simulink model "ISReferenceApplication"  (R2019b)
settings: Solver=VariableStepAuto  StartTime=0.0  StopTime=10.0  RelTol=1e-3
undefined symbols (not defined in the file or in its folder): C_Brake, C_Final, C_Front, C_Middle, C_out_Brake, C_out_Final, C_out_Front, C_out_Middle, Co, Cso, D_out_Brake, D_out_Final, D_out_Front, D_out_Middle, Downshift_Speeds, F, F_Brake, F_Final, F_Front, F_Middle, Fs, G_Brake, G_Final, G_Front, G_Middle, G_sys_Brake, G_sys_Final, G_sys_Front, G_sys_Middle, Gd, Gd_Brake, Gd_Final, Gsd, h, H_Brake, H_Final, H_Front, H_Middle, H_sys_Brake, H_sys_Final, H_sys_Front, H_sys_Middle, Hd, Hd_Brake, Hd_Final, Hsd, JE, JE_Brake, JE_Final, JE_Front, JE_Middle, JEs, JF_part, JF_part_Brake, JF_part_Final, JF_parts, Ld, Ld_Brake, Ld_Final, Ld_Front ... (+21)
libraries: simulink x5, autolibutils x3, sim3dlib x2, vehdynlibviscommon x1
(part 1 of 4)
settings Model: Creator=User  LastModifiedBy=User

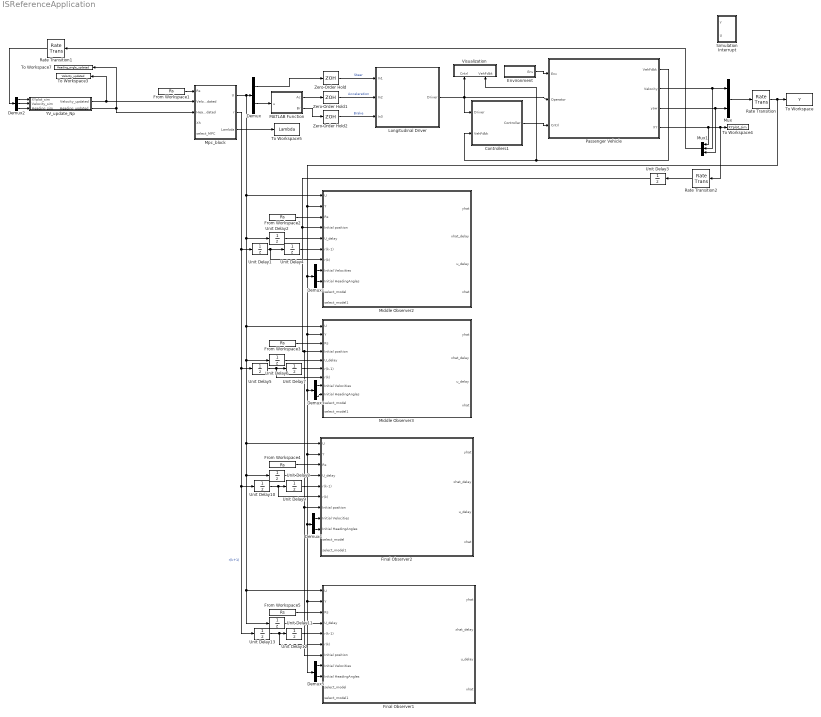
== system ISReferenceApplication ==
  Controllers1 : Subsystem
      mask Display: image('SystemControllers.png')
  Demux{,1,3..5} (5 alike) : Demux  Outputs=2
  Demux2 : Demux  Outputs=3
  Environment : Subsystem  TreatAsAtomicUnit=on
      mask Display: disp('Environment')
  Final Observer1 : Subsystem
  Final Observer2 : Subsystem
  From Workspace{1..5} (5 alike) : FromWorkspace  VariableName=Rs  SampleTime=Ts
  Longitudinal Driver : Subsystem  SystemSampleTime=Tf  VariantControl=0
      mask Display: image('longitudinal_driver_pedals.png');
  MATLAB Function : MATLAB Function  TreatAsAtomicUnit=on  SystemSampleTime=Ts
  Middle Observer2 : Subsystem
  Middle Observer3 : Subsystem
  Mpc_block : Subsystem  TreatAsAtomicUnit=on  SystemSampleTime=Ts
  Mux : Mux  Inputs=2
  Mux1 : Mux  Inputs=3
  Passenger Vehicle : Subsystem
      mask Display: image('PassengerVehicle.png')
  Rate Transition : RateTransition  OutPortSampleTime=Ts
  Rate Transition1 : RateTransition  OutPortSampleTime=Ts
  Rate Transition2 : RateTransition  OutPortSampleTime=Ts
  "Simulation Interrupt " : Subsystem
  To Workspace : ToWorkspace  VariableName=Y  SampleTime=Ts
  To Workspace3 : ToWorkspace  VariableName=Velocity_updated  SampleTime=Ts
      settings: Save2DSignal=2-D array (concatenate along first dimension)
  To Workspace4 : ToWorkspace  VariableName=XYplot_sim  SampleTime=Ts
  To Workspace5 : ToWorkspace  VariableName=Lambda  SampleTime=Ts
  To Workspace7 : ToWorkspace  VariableName=Heading_angle_updated  SampleTime=Ts
      settings: Save2DSignal=2-D array (concatenate along first dimension)
  Unit Delay{1..13} (13 alike) : UnitDelay  SampleTime=Ts  HasFrameUpgradeWarning=on
  Visualization : Subsystem  TreatAsAtomicUnit=on
      mask Display: disp('Visualization')
  YV_update_Np : Subsystem  TreatAsAtomicUnit=on
  Zero-Order Hold : ZeroOrderHold  SampleTime=Tf
  Zero-Order Hold1 : ZeroOrderHold  SampleTime=Tf
  Zero-Order Hold2 : ZeroOrderHold  SampleTime=Tf
  wires:
  Controllers1/1(Controller) -> Passenger Vehicle/3(Cntrl)
  Longitudinal Driver/1(Driver) -> Visualization/1(Cntrl), Controllers1/1(Driver), Passenger Vehicle/2(Operator)
  Environment/1(Env) -> Passenger Vehicle/1(Env)
  Passenger Vehicle/1(VehFdbk) -> Visualization/2(VehFdbk), Controllers1/2(VehFdbk)
  Zero-Order Hold2/1 -> Longitudinal Driver/3(In3)  "Brake"
  Zero-Order Hold1/1 -> Longitudinal Driver/2(In2)  "Acceleration"
  Zero-Order Hold/1 -> Longitudinal Driver/1(In1)  "Steer"
  MATLAB Function/1(Ac) -> Zero-Order Hold1/1
  MATLAB Function/2(Br) -> Zero-Order Hold2/1
  Demux/2 -> MATLAB Function/1(u)
  Demux/1 -> Zero-Order Hold/1
  Mpc_block/1(U) -> Middle Observer2/1(U), Unit Delay11/1, Final Observer1/1(U), Unit Delay8/1, Final Observer2/1(U), Unit Delay6/1, Middle Observer3/1(U), Unit Delay2/1, Demux/1
  Mpc_block/3(Lambda) -> To Workspace5/1
  From Workspace1/1 -> Mpc_block/1(Rs)
  YV_update_Np/1(Velocity_updated) -> To Workspace3/1, Mpc_block/2(Velocity_updated)
  YV_update_Np/2(Heading_updated) -> To Workspace7/1, Mpc_block/3(Heading_updated)
  Demux2/1 -> YV_update_Np/1(XYplot_sim)
  Demux2/2 -> YV_update_Np/2(Velocity_sim)
  Demux2/3 -> YV_update_Np/3(Heading_sim)
  Rate Transition1/1 -> Demux2/1
  Mux/1 -> Rate Transition/1
  Passenger Vehicle/2(Velocity) -> Mux1/2, Mux/1
  Passenger Vehicle/3(yaw) -> Mux1/3, Mux/2
  Passenger Vehicle/4(XY) -> Mux1/1, Rate Transition2/1, To Workspace4/1
  Rate Transition/1 -> Final Observer2/2(Y), Final Observer1/2(Y), Demux5/1, Demux4/1, Demux3/1, Middle Observer3/2(Y), Demux1/1, Middle Observer2/2(Y), To Workspace/1
  Mux1/1 -> Rate Transition1/1
  Rate Transition2/1 -> Unit Delay3/1
  Unit Delay3/1 -> Final Observer1/7(Initial position), Final Observer2/7(Initial position), Middle Observer3/4(Initial position), Middle Observer2/4(Initial position)
  Unit Delay2/1 -> Middle Observer2/5(U_delay)
  Unit Delay4/1 -> Middle Observer2/6(r(k-1))
  Unit Delay1/1 -> Middle Observer2/7(r(k)), Unit Delay4/1
  Mpc_block/2(r) -> Unit Delay13/1, Unit Delay10/1, Unit Delay5/1, Unit Delay1/1  "r(k+1)"
  From Workspace2/1 -> Middle Observer2/3(Rs)
  Demux1/1 -> Middle Observer2/8(Initial Velocities)
  Demux1/2 -> Middle Observer2/9(Initial HeadingAngles)
  Unit Delay6/1 -> Middle Observer3/5(U_delay)
  Unit Delay7/1 -> Middle Observer3/6(r(k-1))
  Unit Delay5/1 -> Middle Observer3/7(r(k)), Unit Delay7/1
  From Workspace3/1 -> Middle Observer3/3(Rs)
  Demux3/1 -> Middle Observer3/8(Initial Velocities)
  Demux3/2 -> Middle Observer3/9(Initial HeadingAngles)
  From Workspace4/1 -> Final Observer2/3(Rs)
  Unit Delay8/1 -> Final Observer2/4(U_delay)
  Unit Delay9/1 -> Final Observer2/5(r(k-1))
  Unit Delay10/1 -> Final Observer2/6(r(k)), Unit Delay9/1
  Demux4/1 -> Final Observer2/8(Initial Velocities)
  Demux4/2 -> Final Observer2/9(Initial HeadingAngles)
  From Workspace5/1 -> Final Observer1/3(Rs)
  Unit Delay11/1 -> Final Observer1/4(U_delay)
  Unit Delay12/1 -> Final Observer1/5(r(k-1))
  Unit Delay13/1 -> Final Observer1/6(r(k)), Unit Delay12/1
  Demux5/1 -> Final Observer1/8(Initial Velocities)
  Demux5/2 -> Final Observer1/9(Initial HeadingAngles)

== system ISReferenceApplication/Controllers1 ==
  Driver : Inport
  VehFdbk : Inport  Port=2
  Active Differential Control : Subsystem  VariantControlMode=Label  Variant=on  LabelModeActiveChoice=0
  Brake Controller : Subsystem
  Bus Creator{,1..2,4} (4 alike) : BusCreator  Inputs=1
  Bus Creator3 : BusCreator  Inputs=4
  Bus Selector : BusSelector  OutputSignals=Body.xdot,Wheels.Kappa,Body.r
  Bus Selector1 : BusSelector  OutputSignals=Driveline.EngSpd,Driveline.PropShftSpd
  Bus Selector2 : BusSelector  OutputSignals=AccelCmd,DecelCmd
  Bus Selector3 : BusSelector  OutputSignals=SteerCmd
  ECU : Subsystem
  Max : MinMax  Function=max  Inputs=2
  Transmission Controller : Subsystem
  Controller : Outport  VectorParamsAs1DForOutWhenUnconnected=off
  wires:
  Bus Selector/3 -> Active Differential Control/1(YawRate)  "<r>"
  [DiffTrqCmd] -> Max/2
  Max/1 -> Bus Creator/1  "EngTrqCmd"
  Active Differential Control/2(TrqCmd) -> [DiffTrqCmd]
  Bus Selector3/1 -> Active Differential Control/2(Steer)  "<SteerCmd>"
  Active Differential Control/1(DiffPrsCmd) -> Bus Creator4/1  "DiffPrsCmd"
  Bus Creator4/1 -> Bus Creator3/4  "Diff"
  Bus Creator3/1 -> Controller/1  "Controller"
  Bus Creator2/1 -> Bus Creator3/3  "Brake"
  Bus Creator1/1 -> Bus Creator3/2  "Transmission"
  Bus Creator/1 -> Bus Creator3/1  "ECU"
  Bus Selector2/2 -> Brake Controller/1(BrkCmd)  "<DecelCmd>"
  Bus Selector2/1 -> ECU/1(<Accel>), Transmission Controller/1(Acc)  "<AccelCmd>"
  Driver/1 -> Bus Selector2/1, Bus Selector3/1
  Bus Selector1/2 -> Transmission Controller/3(PropShaftSpd)  "<PropShftSpd>"
  Bus Selector1/1 -> Transmission Controller/2(EngSpd)  "<EngSpd>"
  Bus Selector/1 -> Brake Controller/2(xdot)  "<xdot>"
  VehFdbk/1 -> Bus Selector1/1, Bus Selector/1
  Brake Controller/1(PCmd) -> Bus Creator2/1  "BrkPrsCmd"
  ECU/1(Trq Cmd) -> Max/1
  Bus Selector/2 -> Brake Controller/3(kappa)  "<Kappa>"
  Transmission Controller/1(Gear) -> Bus Creator1/1  "GearCmd"

== system ISReferenceApplication/Environment ==
  Bus Creator : BusCreator  Inputs=4
  Bus Creator1 : BusCreator  Inputs=2
  Bus Creator2 : BusCreator  Inputs=4
  Bus Creator3 : BusCreator  Inputs=2
  Constant1 : Constant  Value=zeros(4,1)
  Constant3 : Constant  Value=0
  Constant4 : Constant  Value=0
  Constant5 : Constant  Value=0
  Demux : Demux
  Demux1 : Demux
  Friction : Constant  Value=ones(4,1).*1
  Vector Concatenate : Concatenate  NumInputs=3
  Env : Outport  VectorParamsAs1DForOutWhenUnconnected=off
  wires:
  Bus Creator1/1 -> Env/1
  Bus Creator3/1 -> Bus Creator1/2  "Gnd"
  Friction/1 -> Demux1/1
  Demux1/1 -> Bus Creator2/1  "mu_FL"
  Demux1/2 -> Bus Creator2/2  "mu_FR"
  Demux1/4 -> Bus Creator2/4  "mu_RR"
  Demux1/3 -> Bus Creator2/3  "mu_RL"
  Constant4/1 -> Vector Concatenate/2  "Y"
  Demux/4 -> Bus Creator/4  "G_RR_z"
  Constant3/1 -> Vector Concatenate/1  "X"
  Vector Concatenate/1 -> Bus Creator1/1  "Wind"
  Demux/1 -> Bus Creator/1  "G_FL_z"
  Constant5/1 -> Vector Concatenate/3  "Z"
  Demux/3 -> Bus Creator/3  "G_RL_z"
  Demux/2 -> Bus Creator/2  "G_FR_z"
  Bus Creator/1 -> Bus Creator3/1  "z"
  Bus Creator2/1 -> Bus Creator3/2  "mu"
  Constant1/1 -> Demux/1

== system ISReferenceApplication/Final Observer1 ==
  U : Inport
  Y : Inport  Port=2
  Rs : Inport  Port=3
  U_delay : Inport  Port=4
  r(k-1) : Inport  Port=5
  r(k) : Inport  Port=6
  Initial position : Inport  Port=7
  Initial Velocities : Inport  Port=8
  Initial HeadingAngles : Inport  Port=9
  select_model : Inport  Port=10
  select_model1 : Inport  Port=11
  C_Brake2 : Gain  Gain=C_Brake  Multiplication=Matrix(K*u) (u vector)
  Delay : Delay  DelayLength=1  InitialConditionSource=Input port  InitialCondition=0  ExternalReset=Rising  SampleTime=Ts
      settings: InputPortMap=u0,r5,p4
  Delay1 : Delay  DelayLength=1  InitialConditionSource=Input port  InitialCondition=0  ExternalReset=Rising  SampleTime=Ts
      settings: InputPortMap=u0,r5,p4
  Gd_Brake : Gain  Gain=Gd_Brake  Multiplication=Matrix(K*u) (u vector)
  Hd_Brake : Gain  Gain=Hd_Brake  Multiplication=Matrix(K*u) (u vector)
  Ld_Brake1 : Gain  Gain=Ld_Brake  Multiplication=Matrix(K*u) (u vector)
  Ld_Brake2 : Gain  Gain=Ld_Brake  Multiplication=Matrix(K*u) (u vector)
  MATLAB Function1 : MATLAB Function  TreatAsAtomicUnit=on
  Subsystem : Subsystem
  Sum4 : Sum  Inputs=+++
  Switch : Switch  Threshold=4
  Switch1 : Switch  Threshold=4
  yhat : Outport  VectorParamsAs1DForOutWhenUnconnected=off
  xhat_delay : Outport  Port=2  VectorParamsAs1DForOutWhenUnconnected=off
  u_delay : Outport  Port=3  VectorParamsAs1DForOutWhenUnconnected=off
  xhat : Outport  Port=4  VectorParamsAs1DForOutWhenUnconnected=off
  wires:
  Switch/1 -> Delay1/1
  U/1 -> Switch/1
  Gd_Brake/1 -> Sum4/3
  Delay/1 -> Gd_Brake/1, xhat_delay/1
  Ld_Brake1/1 -> Sum4/1
  Hd_Brake/1 -> Sum4/2
  C_Brake2/1 -> yhat/1
  Delay1/1 -> u_delay/1, Hd_Brake/1
  Sum4/1 -> Subsystem/8(Xh_sim), xhat/1, C_Brake2/1, Delay/1
  Y/1 -> Switch1/1
  Switch1/1 -> Ld_Brake1/1
  r(k-1)/1 -> Ld_Brake2/1, Subsystem/6(r(k-1))
  Ld_Brake2/1 -> Delay/3
  r(k)/1 -> Subsystem/7(r(k))
  Rs/1 -> Subsystem/1(Rs)
  U_delay/1 -> Delay1/3, Subsystem/2(U_delay)
  Initial position/1 -> Subsystem/3(Initial position)
  Initial Velocities/1 -> Subsystem/4(Initial Velocities)
  Initial HeadingAngles/1 -> Subsystem/5(Initial HeadingAngles)
  Subsystem/1(Y) -> Switch1/3
  Subsystem/2(U) -> Switch/3
  MATLAB Function1/1(tri) -> Delay/2, Delay1/2
  select_model/1 -> MATLAB Function1/1(select_model), Subsystem/9(select_model)
  select_model1/1 -> Switch/2, Switch1/2

== system ISReferenceApplication/Final Observer2 ==
  U : Inport
  Y : Inport  Port=2
  Rs : Inport  Port=3
  U_delay : Inport  Port=4
  r(k-1) : Inport  Port=5
  r(k) : Inport  Port=6
  Initial position : Inport  Port=7
  Initial Velocities : Inport  Port=8
  Initial HeadingAngles : Inport  Port=9
  select_model : Inport  Port=10
  select_model1 : Inport  Port=11
  C_Final2 : Gain  Gain=C_Final  Multiplication=Matrix(K*u) (u vector)
  Delay : Delay  DelayLength=1  InitialConditionSource=Input port  InitialCondition=0  ExternalReset=Rising  SampleTime=Ts
      settings: InputPortMap=u0,r5,p4
  Delay1 : Delay  DelayLength=1  InitialConditionSource=Input port  InitialCondition=0  ExternalReset=Rising  SampleTime=Ts
      settings: InputPortMap=u0,r5,p4
  Gd_Final : Gain  Gain=Gd_Final  Multiplication=Matrix(K*u) (u vector)
  Hd_Final : Gain  Gain=Hd_Final  Multiplication=Matrix(K*u) (u vector)
  Ld_Final1 : Gain  Gain=Ld_Final  Multiplication=Matrix(K*u) (u vector)
  Ld_Final2 : Gain  Gain=Ld_Final  Multiplication=Matrix(K*u) (u vector)
  MATLAB Function1 : MATLAB Function  TreatAsAtomicUnit=on
  Subsystem : Subsystem
  Sum4 : Sum  Inputs=+++
  Switch : Switch  Threshold=3
  Switch1 : Switch  Threshold=3
  yhat : Outport  VectorParamsAs1DForOutWhenUnconnected=off
  xhat_delay : Outport  Port=2  VectorParamsAs1DForOutWhenUnconnected=off
  u_delay : Outport  Port=3  VectorParamsAs1DForOutWhenUnconnected=off
  xhat : Outport  Port=4  VectorParamsAs1DForOutWhenUnconnected=off
  wires:
  select_model1/1 -> Switch1/2, Switch/2
  select_model/1 -> Subsystem/9(select_model), MATLAB Function1/1(select_model)
  MATLAB Function1/1(tri) -> Delay1/2, Delay/2
  Subsystem/2(U) -> Switch/3
  Subsystem/1(Y) -> Switch1/3
  Initial HeadingAngles/1 -> Subsystem/5(Initial HeadingAngles)
  Initial Velocities/1 -> Subsystem/4(Initial Velocities)
  Initial position/1 -> Subsystem/3(Initial position)
  U_delay/1 -> Subsystem/2(U_delay), Delay1/3
  Rs/1 -> Subsystem/1(Rs)
  r(k)/1 -> Subsystem/7(r(k))
  Ld_Final2/1 -> Delay/3
  r(k-1)/1 -> Subsystem/6(r(k-1)), Ld_Final2/1
  Y/1 -> Switch1/1, Ld_Final1/1
  Sum4/1 -> Delay/1, C_Final2/1, xhat/1, Subsystem/8(Xh_sim)
  Delay1/1 -> Hd_Final/1, u_delay/1
  C_Final2/1 -> yhat/1
  Hd_Final/1 -> Sum4/2
  Ld_Final1/1 -> Sum4/1
  Delay/1 -> xhat_delay/1, Gd_Final/1
  Gd_Final/1 -> Sum4/3
  U/1 -> Switch/1, Delay1/1

== system ISReferenceApplication/Longitudinal Driver ==
  In1 : Inport  SampleTime=Tf
  In2 : Inport  Port=2  SampleTime=Tf
  In3 : Inport  Port=3  SampleTime=Tf
  Bus Creator1 : BusCreator  Inputs=3
  To Workspace : ToWorkspace  VariableName=Brake  SampleTime=Tf
  To Workspace1 : ToWorkspace  VariableName=Steer  SampleTime=-1
  To Workspace2 : ToWorkspace  VariableName=Acceleration  SampleTime=Tf
  Driver : Outport  VectorParamsAs1DForOutWhenUnconnected=off
  wires:
  In1/1 -> Bus Creator1/1, To Workspace1/1  "Steer"
  In3/1 -> To Workspace/1, Bus Creator1/3  "Brake"
  In2/1 -> Bus Creator1/2, To Workspace2/1  "Accel"
  Bus Creator1/1 -> Driver/1

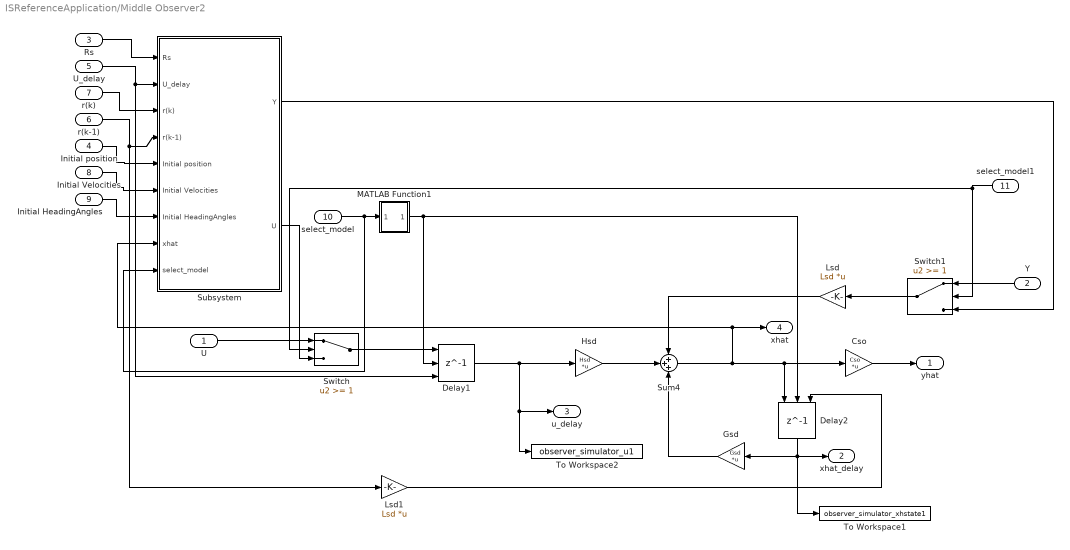
== system ISReferenceApplication/Middle Observer2 ==
  U : Inport
  Y : Inport  Port=2
  Rs : Inport  Port=3
  Initial position : Inport  Port=4
  U_delay : Inport  Port=5
  r(k-1) : Inport  Port=6
  r(k) : Inport  Port=7
  Initial Velocities : Inport  Port=8
  Initial HeadingAngles : Inport  Port=9
  select_model : Inport  Port=10
  select_model1 : Inport  Port=11
  Cso : Gain  Gain=Cso  Multiplication=Matrix(K*u) (u vector)
  Delay1 : Delay  DelayLength=1  InitialConditionSource=Input port  InitialCondition=0  ExternalReset=Rising  SampleTime=Ts
      settings: InputPortMap=u0,r5,p4
  Delay2 : Delay  DelayLength=1  InitialConditionSource=Input port  InitialCondition=0  ExternalReset=Rising  SampleTime=Ts
      settings: InputPortMap=u0,r5,p4
  Gsd : Gain  Gain=Gsd  Multiplication=Matrix(K*u) (u vector)
  Hsd : Gain  Gain=Hsd  Multiplication=Matrix(K*u) (u vector)
  Lsd : Gain  Gain=Lsd  Multiplication=Matrix(K*u) (u vector)
  Lsd1 : Gain  Gain=Lsd  Multiplication=Matrix(K*u) (u vector)
  MATLAB Function1 : MATLAB Function  TreatAsAtomicUnit=on
  Subsystem : Subsystem
  Sum4 : Sum  Inputs=+++
  Switch : Switch  Threshold=1
  Switch1 : Switch  Threshold=1
  To Workspace1 : ToWorkspace  VariableName=observer_simulator_xhstate1  SampleTime=Ts
  To Workspace2 : ToWorkspace  VariableName=observer_simulator_u1  SampleTime=Ts
  yhat : Outport  VectorParamsAs1DForOutWhenUnconnected=off
  xhat_delay : Outport  Port=2  VectorParamsAs1DForOutWhenUnconnected=off
  u_delay : Outport  Port=3  VectorParamsAs1DForOutWhenUnconnected=off
  xhat : Outport  Port=4  VectorParamsAs1DForOutWhenUnconnected=off
  wires:
  select_model1/1 -> Switch1/2, Switch/2
  MATLAB Function1/1(tri) -> Delay1/2, Delay2/2
  select_model/1 -> MATLAB Function1/1(select_model), Subsystem/9(select_model)
  Switch/1 -> Delay1/1
  Initial HeadingAngles/1 -> Subsystem/7(Initial HeadingAngles)
  Initial Velocities/1 -> Subsystem/6(Initial Velocities)
  r(k)/1 -> Subsystem/3(r(k))
  U_delay/1 -> Subsystem/2(U_delay), Delay1/3
  r(k-1)/1 -> Subsystem/4(r(k-1)), Lsd1/1
  Subsystem/1(Y) -> Switch1/3
  Subsystem/2(U) -> Switch/3
  Initial position/1 -> Subsystem/5(Initial position)
  Rs/1 -> Subsystem/1(Rs)
  Switch1/1 -> Lsd/1
  Y/1 -> Switch1/1
  Lsd1/1 -> Delay2/3
  U/1 -> Switch/1
  Delay2/1 -> xhat_delay/1, Gsd/1, To Workspace1/1
  Lsd/1 -> Sum4/1
  Gsd/1 -> Sum4/3
  Hsd/1 -> Sum4/2
  Cso/1 -> yhat/1
  Sum4/1 -> Delay2/1, Cso/1, Subsystem/8(xhat), xhat/1
  Delay1/1 -> Hsd/1, To Workspace2/1, u_delay/1

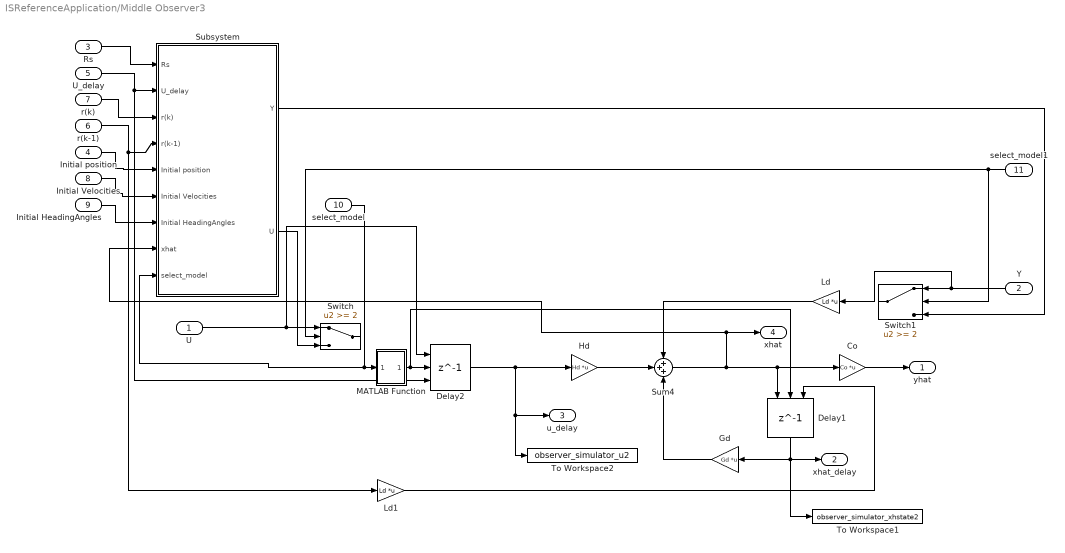
== system ISReferenceApplication/Middle Observer3 ==
  U : Inport
  Y : Inport  Port=2
  Rs : Inport  Port=3
  Initial position : Inport  Port=4
  U_delay : Inport  Port=5
  r(k-1) : Inport  Port=6
  r(k) : Inport  Port=7
  Initial Velocities : Inport  Port=8
  Initial HeadingAngles : Inport  Port=9
  select_model : Inport  Port=10
  select_model1 : Inport  Port=11
  Co : Gain  Gain=Co  Multiplication=Matrix(K*u) (u vector)
  Delay1 : Delay  DelayLength=1  InitialConditionSource=Input port  InitialCondition=0  ExternalReset=Rising  SampleTime=Ts
      settings: InputPortMap=u0,r5,p4
  Delay2 : Delay  DelayLength=1  InitialConditionSource=Input port  InitialCondition=0  ExternalReset=Rising  SampleTime=Ts
      settings: InputPortMap=u0,r5,p4
  Gd : Gain  Gain=Gd  Multiplication=Matrix(K*u) (u vector)
  Hd : Gain  Gain=Hd  Multiplication=Matrix(K*u) (u vector)
  Ld : Gain  Gain=Ld  Multiplication=Matrix(K*u) (u vector)
  Ld1 : Gain  Gain=Ld  Multiplication=Matrix(K*u) (u vector)
  MATLAB Function : MATLAB Function  TreatAsAtomicUnit=on
  Subsystem : Subsystem
  Sum4 : Sum  Inputs=+++
  Switch : Switch  Threshold=2
  Switch1 : Switch  Threshold=2
  To Workspace1 : ToWorkspace  VariableName=observer_simulator_xhstate2  SampleTime=Ts
  To Workspace2 : ToWorkspace  VariableName=observer_simulator_u2  SampleTime=Ts
  yhat : Outport  VectorParamsAs1DForOutWhenUnconnected=off
  xhat_delay : Outport  Port=2  VectorParamsAs1DForOutWhenUnconnected=off
  u_delay : Outport  Port=3  VectorParamsAs1DForOutWhenUnconnected=off
  xhat : Outport  Port=4  VectorParamsAs1DForOutWhenUnconnected=off
  wires:
  select_model1/1 -> Switch1/2, Switch/2
  MATLAB Function/1(tri) -> Delay1/2, Delay2/2
  select_model/1 -> MATLAB Function/1(select_model), Subsystem/9(select_model)
  Delay2/1 -> u_delay/1, To Workspace2/1, Hd/1
  Sum4/1 -> xhat/1, Subsystem/8(xhat), Co/1, Delay1/1
  Co/1 -> yhat/1
  Hd/1 -> Sum4/2
  Gd/1 -> Sum4/3
  Ld/1 -> Sum4/1
  Delay1/1 -> To Workspace1/1, Gd/1, xhat_delay/1
  U/1 -> Switch/1, Delay2/1
  Ld1/1 -> Delay1/3
  Y/1 -> Switch1/1, Ld/1
  Rs/1 -> Subsystem/1(Rs)
  Initial position/1 -> Subsystem/5(Initial position)
  Subsystem/2(U) -> Switch/3
  Subsystem/1(Y) -> Switch1/3
  r(k-1)/1 -> Ld1/1, Subsystem/4(r(k-1))
  U_delay/1 -> Subsystem/2(U_delay), Delay2/3
  r(k)/1 -> Subsystem/3(r(k))
  Initial Velocities/1 -> Subsystem/6(Initial Velocities)
  Initial HeadingAngles/1 -> Subsystem/7(Initial HeadingAngles)

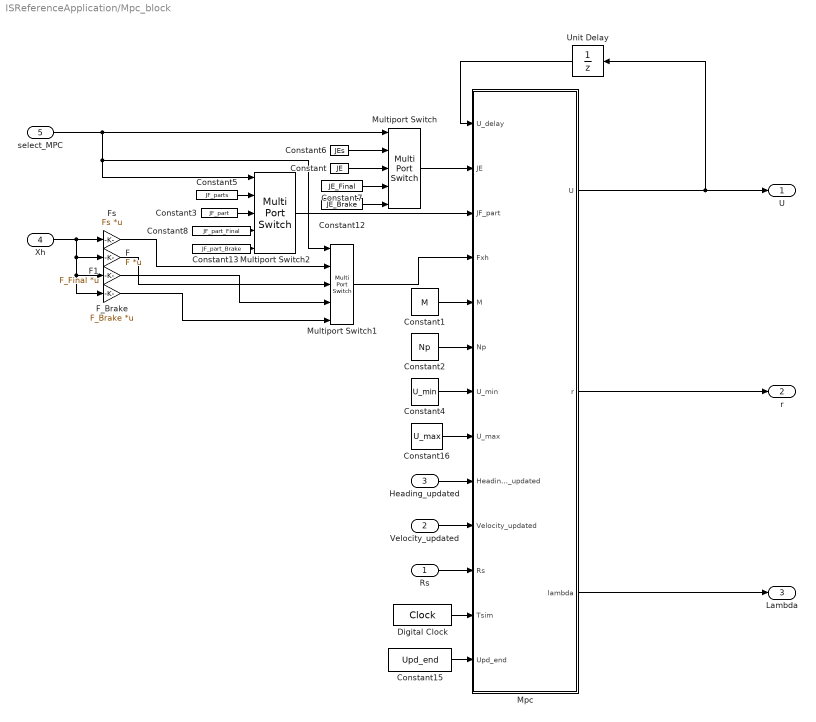
== system ISReferenceApplication/Mpc_block ==
  Rs : Inport  SampleTime=Ts  LockScale=on
  Velocity_updated : Inport  Port=2  SampleTime=Ts
  Heading_updated : Inport  Port=3  SampleTime=Ts  LockScale=on
  Xh : Inport  Port=4
  select_MPC : Inport  Port=5
  Constant : Constant  Value=JE  VectorParams1D=off  SampleTime=-1
  Constant1 : Constant  Value=M  VectorParams1D=off  SampleTime=-1
  Constant12 : Constant  Value=JE_Brake  VectorParams1D=off  SampleTime=-1
  Constant13 : Constant  Value=JF_part_Brake  VectorParams1D=off  SampleTime=-1
  Constant15 : Constant  Value=Upd_end  VectorParams1D=off  SampleTime=-1
  Constant16 : Constant  Value=U_max  VectorParams1D=off  SampleTime=-1
  Constant2 : Constant  Value=Np  SampleTime=-1
  Constant3 : Constant  Value=JF_part  VectorParams1D=off  SampleTime=-1
  Constant4 : Constant  Value=U_min  VectorParams1D=off  SampleTime=-1
  Constant5 : Constant  Value=JF_parts  VectorParams1D=off  SampleTime=-1
  Constant6 : Constant  Value=JEs  VectorParams1D=off  SampleTime=-1
  Constant7 : Constant  Value=JE_Final  VectorParams1D=off  SampleTime=-1
  Constant8 : Constant  Value=JF_part_Final  VectorParams1D=off  SampleTime=-1
  Digital Clock : DigitalClock  SampleTime=Ts
  F : Gain  Gain=F  Multiplication=Matrix(K*u) (u vector)
  F1 : Gain  Gain=F_Final  Multiplication=Matrix(K*u) (u vector)
  F_Brake : Gain  Gain=F_Brake  Multiplication=Matrix(K*u) (u vector)
  Fs : Gain  Gain=Fs  Multiplication=Matrix(K*u) (u vector)
  Mpc : MATLAB Function  TreatAsAtomicUnit=on  SystemSampleTime=Ts
  Multiport Switch : MultiPortSwitch  Inputs=4
  Multiport Switch1 : MultiPortSwitch  Inputs=4
  Multiport Switch2 : MultiPortSwitch  Inputs=4
  Unit Delay : UnitDelay  InitialCondition=[0;0]  SampleTime=Ts  HasFrameUpgradeWarning=on
  U : Outport  VectorParamsAs1DForOutWhenUnconnected=off
  r : Outport  Port=2  VectorParamsAs1DForOutWhenUnconnected=off
  Lambda : Outport  Port=3  VectorParamsAs1DForOutWhenUnconnected=off
  wires:
  Heading_updated/1 -> Mpc/9(Heading_updated)
  Velocity_updated/1 -> Mpc/10(Velocity_updated)
  Mpc/3(lambda) -> Lambda/1
  Constant16/1 -> Mpc/8(U_max)
  Digital Clock/1 -> Mpc/12(Tsim)
  Constant15/1 -> Mpc/13(Upd_end)
  Mpc/2(r) -> r/1
  F_Brake/1 -> Multiport Switch1/5
  Constant13/1 -> Multiport Switch2/5
  Constant12/1 -> Multiport Switch/5
  Constant8/1 -> Multiport Switch2/4
  Constant7/1 -> Multiport Switch/4
  F1/1 -> Multiport Switch1/4
  Constant6/1 -> Multiport Switch/2
  Constant/1 -> Multiport Switch/3
  select_MPC/1 -> Multiport Switch/1, Multiport Switch1/1, Multiport Switch2/1
  Constant4/1 -> Mpc/7(U_min)
  Multiport Switch/1 -> Mpc/2(JE)
  Fs/1 -> Multiport Switch1/2
  F/1 -> Multiport Switch1/3
  Constant5/1 -> Multiport Switch2/2
  Constant3/1 -> Multiport Switch2/3
  Multiport Switch2/1 -> Mpc/3(JF_part)
  Multiport Switch1/1 -> Mpc/4(Fxh)
  Rs/1 -> Mpc/11(Rs)
  Xh/1 -> Fs/1, F/1, F1/1, F_Brake/1
  Constant2/1 -> Mpc/6(Np)
  Mpc/1(U) -> U/1, Unit Delay/1
  Constant1/1 -> Mpc/5(M)
  Unit Delay/1 -> Mpc/1(U_delay)

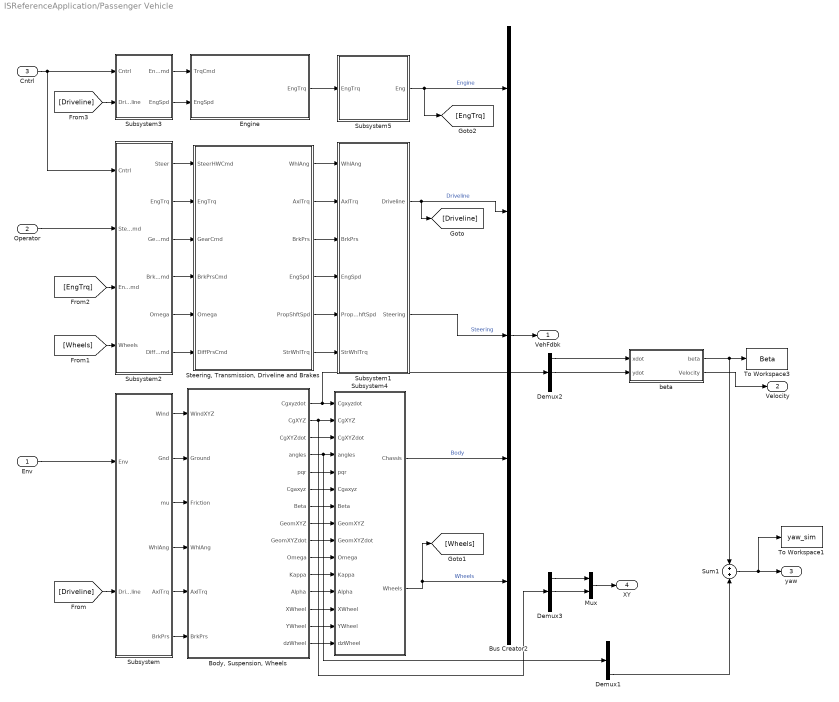
== system ISReferenceApplication/Passenger Vehicle ==
  Env : Inport
  Operator : Inport  Port=2
  Cntrl : Inport  Port=3
  "Body, Suspension, Wheels" : Subsystem  VariantControlMode=Label  Variant=on  LabelModeActiveChoice=3
  Bus Creator2 : BusCreator  Inputs=5
  Demux1 : Demux  Outputs=3
  Demux2 : Demux  Outputs=3
  Demux3 : Demux  Outputs=3
  Engine : Subsystem  VariantControlMode=Label  Variant=on  LabelModeActiveChoice=0
  Mux : Mux  Inputs=2
  "Steering, Transmission, Driveline and Brakes" : Subsystem  VariantControlMode=Label  Variant=on  LabelModeActiveChoice=0
  Subsystem : Subsystem
  Subsystem1 : Subsystem
  Subsystem2 : Subsystem
  Subsystem3 : Subsystem
  Subsystem4 : Subsystem
  Subsystem5 : Subsystem
  Sum1 : Sum
  To Workspace1 : ToWorkspace  VariableName=yaw_sim  SampleTime=Ts
  To Workspace3 : ToWorkspace  VariableName=Beta  SampleTime=Ts
  beta : MATLAB Function  TreatAsAtomicUnit=on  SystemSampleTime=Tf
      settings: MinAlgLoopOccurrences=on
  VehFdbk : Outport  VectorParamsAs1DForOutWhenUnconnected=off
  Velocity : Outport  Port=2  VectorParamsAs1DForOutWhenUnconnected=off
  yaw : Outport  Port=3  VectorParamsAs1DForOutWhenUnconnected=off
  XY : Outport  Port=4  VectorParamsAs1DForOutWhenUnconnected=off
  wires:
  "Body, Suspension, Wheels"/12(Alpha) -> Subsystem4/12(Alpha)
  "Body, Suspension, Wheels"/10(Omega) -> Subsystem4/10(Omega)
  "Body, Suspension, Wheels"/9(GeomXYZdot) -> Subsystem4/9(GeomXYZdot)
  "Body, Suspension, Wheels"/2(CgXYZ) -> Demux3/1, Subsystem4/2(CgXYZ)
  "Body, Suspension, Wheels"/13(XWheel) -> Subsystem4/13(XWheel)
  "Body, Suspension, Wheels"/11(Kappa) -> Subsystem4/11(Kappa)
  "Body, Suspension, Wheels"/4(angles) -> Demux1/1, Subsystem4/4(angles)
  "Body, Suspension, Wheels"/8(GeomXYZ) -> Subsystem4/8(GeomXYZ)
  "Body, Suspension, Wheels"/6(Cgaxyz) -> Subsystem4/6(Cgaxyz)
  "Body, Suspension, Wheels"/7(Beta) -> Subsystem4/7(Beta)
  "Body, Suspension, Wheels"/14(YWheel) -> Subsystem4/14(YWheel)
  "Body, Suspension, Wheels"/5(pqr) -> Subsystem4/5(pqr)
  "Body, Suspension, Wheels"/1(Cgxyzdot) -> Demux2/1, Subsystem4/1(Cgxyzdot)
  "Body, Suspension, Wheels"/3(CgXYZdot) -> Subsystem4/3(CgXYZdot)
  "Body, Suspension, Wheels"/15(dzWheel) -> Subsystem4/15(dzWheel)
  Subsystem1/2(Steering) -> Bus Creator2/3  "Steering"
  "Steering, Transmission, Driveline and Brakes"/6(StrWhlTrq) -> Subsystem1/6(StrWhlTrq)
  Subsystem2/6(DiffPrsCmd) -> "Steering, Transmission, Driveline and Brakes"/6(DiffPrsCmd)
  [Driveline] -> Subsystem3/2(Driveline)
  [EngTrq] -> Subsystem2/3(EngTrqCmd)
  [Wheels] -> Subsystem2/4(Wheels)
  [Driveline] -> Subsystem/2(Driveline)
  Subsystem5/1(Eng) -> [EngTrq], Bus Creator2/1  "Engine"
  Subsystem4/2(Wheels) -> Bus Creator2/5, [Wheels]  "Wheels"
  Subsystem4/1(Chassis) -> Bus Creator2/4  "Body"
  Subsystem3/2(EngSpd) -> Engine/2(EngSpd)
  Subsystem3/1(EngTrqCmd) -> Engine/1(TrqCmd)
  Subsystem2/2(EngTrq) -> "Steering, Transmission, Driveline and Brakes"/2(EngTrq)
  Engine/1(EngTrq) -> Subsystem5/1("EngTrq ")
  Subsystem2/5(Omega) -> "Steering, Transmission, Driveline and Brakes"/5(Omega)
  Subsystem2/4(BrkPrsCmd) -> "Steering, Transmission, Driveline and Brakes"/4(BrkPrsCmd)
  Subsystem2/3(GearCmd) -> "Steering, Transmission, Driveline and Brakes"/3(GearCmd)
  Subsystem2/1(Steer) -> "Steering, Transmission, Driveline and Brakes"/1(SteerHWCmd)
  Cntrl/1 -> Subsystem2/1(Cntrl), Subsystem3/1(Cntrl)
  Operator/1 -> Subsystem2/2(SteerCmd)
  "Steering, Transmission, Driveline and Brakes"/5(PropShftSpd) -> Subsystem1/5(PropShftSpd)
  "Steering, Transmission, Driveline and Brakes"/4(EngSpd) -> Subsystem1/4(EngSpd)
  "Steering, Transmission, Driveline and Brakes"/3(BrkPrs) -> Subsystem1/3(BrkPrs)
  "Steering, Transmission, Driveline and Brakes"/2(AxlTrq) -> Subsystem1/2(AxlTrq)
  "Steering, Transmission, Driveline and Brakes"/1(WhlAng) -> Subsystem1/1(WhlAng)
  Subsystem1/1(Driveline) -> Bus Creator2/2, [Driveline]  "Driveline"
  Subsystem/6(BrkPrs) -> "Body, Suspension, Wheels"/6(BrkPrs)
  Subsystem/5(AxlTrq) -> "Body, Suspension, Wheels"/5(AxlTrq)
  Subsystem/4(WhlAng) -> "Body, Suspension, Wheels"/4(WhlAng)
  Subsystem/3(mu) -> "Body, Suspension, Wheels"/3(Friction)
  Subsystem/2(Gnd) -> "Body, Suspension, Wheels"/2(Ground)
  Subsystem/1(Wind) -> "Body, Suspension, Wheels"/1(WindXYZ)
  Env/1 -> Subsystem/1(Env)
  Bus Creator2/1 -> VehFdbk/1
  Demux2/1 -> beta/1(xdot)
  Demux2/2 -> beta/2(ydot)
  beta/1(beta) -> Sum1/1, To Workspace3/1
  beta/2(Velocity) -> Velocity/1
  Demux1/3 -> Sum1/2
  Sum1/1 -> To Workspace1/1, yaw/1
  Mux/1 -> XY/1
  Demux3/1 -> Mux/1
  Demux3/2 -> Mux/2

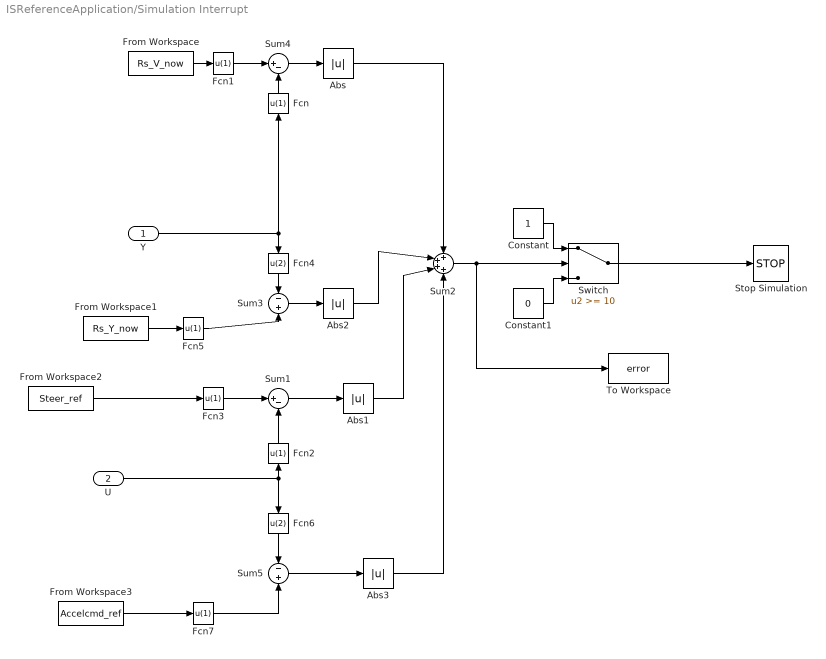
== system ISReferenceApplication/Simulation Interrupt  ==
  Y : Inport
  U : Inport  Port=2
  Abs{,1..3} (4 alike) : Abs
  Constant : Constant
  Constant1 : Constant  Value=0
  Fcn{,1..3,5,7} (6 alike) : Fcn  Expr=u(1)
  Fcn4 : Fcn  Expr=u(2)
  Fcn6 : Fcn  Expr=u(2)
  From Workspace : FromWorkspace  VariableName=Rs_V_now  SampleTime=Ts
  From Workspace1 : FromWorkspace  VariableName=Rs_Y_now  SampleTime=Ts
  From Workspace2 : FromWorkspace  VariableName=Steer_ref  SampleTime=Ts
  From Workspace3 : FromWorkspace  VariableName=Accelcmd_ref  SampleTime=Ts
  Stop Simulation : Stop
  Sum1 : Sum  Inputs=|+-
  Sum2 : Sum  Inputs=++++
  Sum3 : Sum  Inputs=-+
  Sum4 : Sum  Inputs=|+-
  Sum5 : Sum  Inputs=-+
  Switch : Switch  Threshold=10
  To Workspace : ToWorkspace  VariableName=error  SaveFormat=Timeseries  SampleTime=Ts
  wires:
  Abs2/1 -> Sum2/2
  Sum3/1 -> Abs2/1
  Abs3/1 -> Sum2/4
  Sum5/1 -> Abs3/1
  Fcn7/1 -> Sum5/2
  From Workspace3/1 -> Fcn7/1
  Fcn6/1 -> Sum5/1
  Fcn4/1 -> Sum3/1
  Sum2/1 -> Switch/2, To Workspace/1
  Fcn5/1 -> Sum3/2
  From Workspace1/1 -> Fcn5/1
  Abs1/1 -> Sum2/3
  Abs/1 -> Sum2/1
  Sum1/1 -> Abs1/1
  Fcn2/1 -> Sum1/2
  Fcn3/1 -> Sum1/1
  From Workspace2/1 -> Fcn3/1
  U/1 -> Fcn2/1, Fcn6/1
  Switch/1 -> Stop Simulation/1
  Constant/1 -> Switch/1
  Constant1/1 -> Switch/3
  Sum4/1 -> Abs/1
  Fcn1/1 -> Sum4/1
  Y/1 -> Fcn4/1, Fcn/1
  Fcn/1 -> Sum4/2
  From Workspace/1 -> Fcn1/1

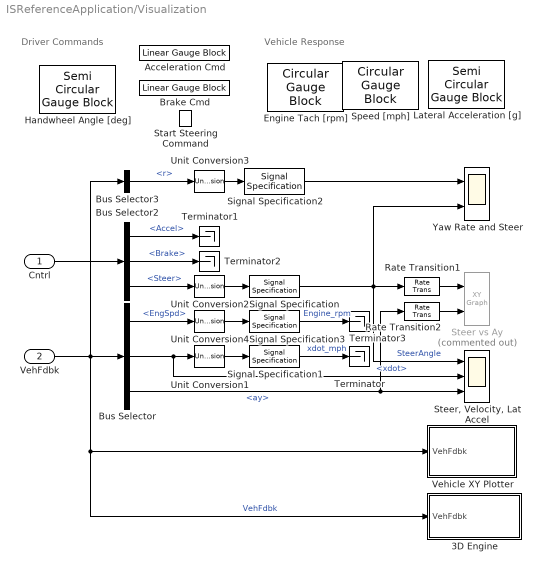
== system ISReferenceApplication/Visualization ==
  note: Vehicle Response
  note: Driver Commands
  Cntrl : Inport
  VehFdbk : Inport  Port=2
  3D Engine : Subsystem  VariantControlMode=Label  Variant=on  LabelModeActiveChoice=0  mask(3D Engine){engine3D=Disabled, SceneDesc=Straight road, dt3D=.03}
      mask prompts: engine3D "3D Engine"; SceneDesc "Scene Description:"; dt3D "Engine frame rate, dt3D [s]:"
      mask help: This subsystem contains the interface blocks which permit the display of the vehicle in 3D virtual environment. Enable it to view the simulation progress, disable it to inhibit the display.
      mask init:
      | switch get_param(gcb,'engine3D')
      |     case 'Disabled'
      |         set_param(gcb,'OverrideUsingVariant','0')
      |     case 'Enabled'
      |        set_param(gcb,'OverrideUsingVariant','1')
      |     otherwise
      |        set_param(gcb,'OverrideUsingVariant','0')
      | end
      settings: AttributesFormatString=%<engine3D>
      mask Help: eval('vdynblkshelp(''vdynblksscenecameraray'')');
      mask TypeOptions engine3D: Enabled | Disabled
      mask Callback engine3D:
      | switch get_param(gcb,'engine3D')
      |     case 'Disabled'
      |         set_param(gcb,'OverrideUsingVariant','0')
      |     case 'Enabled'
      |        set_param(gcb,'OverrideUsingVariant','1')
      |     otherwise
      |        set_param(gcb,'OverrideUsingVariant','0')
      | end
      mask TypeOptions SceneDesc:
      | 3D Engine/Simulation 3D Engine
      | 1/SceneDesc
      mask Display: disp('3D Engine')
  Acceleration Cmd : LinearGaugeBlock  ScaleMax=1
  Brake Cmd : LinearGaugeBlock  ScaleMax=1
  Bus Selector : BusSelector  OutputSignals=Driveline.EngSpd,Body.xdot,Body.ay
  Bus Selector2 : BusSelector  OutputSignals=Accel,Brake,Steer
  Bus Selector3 : BusSelector  OutputSignals=Body.r
  Engine Tach [rpm] : CircularGaugeBlock  ScaleMax=8000  TickInterval=1000
  Handwheel Angle [deg] : SemiCircularGaugeBlock  ScaleMin=-300  ScaleMax=300  TickInterval=60
  Lateral Acceleration [g] : SemiCircularGaugeBlock  ScaleMin=-1  ScaleMax=1  TickInterval=0.5
  Rate Transition1 : RateTransition
  Rate Transition2 : RateTransition
  Signal Specification : SignalSpecification  Unit=deg
  Signal Specification1 : SignalSpecification  Unit=mph
  Signal Specification2 : SignalSpecification  Unit=deg/s
  Signal Specification3 : SignalSpecification  Unit=rpm
  Speed [mph] : CircularGaugeBlock
  Start Steering Command : LampBlock  LabelPosition=Hide
  Steer vs Ay : simulink/Sinks/XY Graph  Commented=on  xmin=-300  xmax=300  ymin=-1.5  ymax=1.5  st=.1
  "Steer, Velocity, Lat Accel" : Scope  NumInputPorts=3
  Terminator{,1..3} (4 alike) : Terminator
  Unit Conversion{1..4} (4 alike) : UnitConversion
  Vehicle XY Plotter : Subsystem  mask(Vehicle XY Plotter){a=VEH.FrontAxlePositionfromCG, b=VEH.RearAxlePositionfromCG, w=VEH.TrackWidth, bufferSize=1024, pltDT=0.1}
      mask prompts: a "Distance to front axle from CG, a [m]:"; b "Distance to rear axle from CG, b [m]:"; w "Track width, w [m]:"; bufferSize "Path buffer sampe size, bufferSize []:"; pltDT "Plot update rate, pltDT [s]:"
      mask help: This block will display a MATLAB figure which indicates the vehicle path, current position and heading velocity.
      mask TypeOptions a: Vehicle XY Plotter/a
      mask TypeOptions b: Vehicle XY Plotter/b
      mask TypeOptions w: Vehicle XY Plotter/w
      mask TypeOptions bufferSize: Vehicle XY Plotter/bufferSize
  Yaw Rate and Steer : Scope  NumInputPorts=2
  wires:
  Bus Selector2/2 -> Terminator2/1  "<Brake>"
  Bus Selector/1 -> Unit Conversion4/1  "<EngSpd>"
  Rate Transition2/1 -> Steer vs Ay/2
  Cntrl/1 -> Bus Selector2/1
  VehFdbk/1 -> 3D Engine/1(VehFdbk), Vehicle XY Plotter/1(VehFdbk), Bus Selector/1, Bus Selector3/1  "VehFdbk"
  Bus Selector/2 -> Unit Conversion1/1, "Steer, Velocity, Lat Accel"/2  "<xdot>"
  Unit Conversion2/1 -> Signal Specification/1
  Rate Transition1/1 -> Steer vs Ay/1
  Bus Selector2/1 -> Terminator1/1  "<Accel>"
  Bus Selector/3 -> "Steer, Velocity, Lat Accel"/3, Rate Transition2/1  "<ay>"
  Unit Conversion1/1 -> Signal Specification1/1
  Signal Specification1/1 -> Terminator/1  "xdot_mph"
  Bus Selector2/3 -> Unit Conversion2/1  "<Steer>"
  Signal Specification/1 -> "Steer, Velocity, Lat Accel"/1, Rate Transition1/1, Yaw Rate and Steer/2  "SteerAngle"
  Signal Specification3/1 -> Terminator3/1  "Engine_rpm"
  Unit Conversion4/1 -> Signal Specification3/1
  Signal Specification2/1 -> Yaw Rate and Steer/1
  Bus Selector3/1 -> Unit Conversion3/1  "<r>"
  Unit Conversion3/1 -> Signal Specification2/1

== system ISReferenceApplication/YV_update_Np ==
  XYplot_sim : Inport
  Velocity_sim : Inport  Port=2
  Heading_sim : Inport  Port=3
  From Workspace1 : FromWorkspace  VariableName=T_sim  SampleTime=Ts
  From Workspace3 : FromWorkspace  VariableName=XY_Ref_Upd  SampleTime=Ts
  MATLAB Function2 : MATLAB Function  TreatAsAtomicUnit=on  SystemSampleTime=Ts
  Velocity_updated : Outport  VectorParamsAs1DForOutWhenUnconnected=off
  Heading_updated : Outport  Port=2  VectorParamsAs1DForOutWhenUnconnected=off
  wires:
  Heading_sim/1 -> MATLAB Function2/4(Yaw_sim)
  Velocity_sim/1 -> MATLAB Function2/3(Velocity_sim)
  XYplot_sim/1 -> MATLAB Function2/2(XYplot_sim)
  From Workspace1/1 -> MATLAB Function2/5(Tsim)
  MATLAB Function2/2(Heading_updated) -> Heading_updated/1
  From Workspace3/1 -> MATLAB Function2/1(XY_ref)
  MATLAB Function2/1(Velocity_updated) -> Velocity_updated/1

== system ISReferenceApplication/Controllers1/Active Differential Control ==
  note: 1) Add Subsystem or Model blocks as valid variant choices.
      | 2) You cannot connect blocks at this level. At simulation, connectivity is automatically
      | determined, based on the active variant and port name matching.
  YawRate : Inport
  Steer : Inport  Port=2
  No Control : Subsystem  VariantControl=0
  Rear Diff Controller : Subsystem  VariantControl=1
  DiffPrsCmd : Outport  VectorParamsAs1DForOutWhenUnconnected=off
  TrqCmd : Outport  Port=2  VectorParamsAs1DForOutWhenUnconnected=off

== system ISReferenceApplication/Controllers1/Brake Controller ==
  BrkCmd : Inport
  xdot : Inport  Port=2
  kappa : Inport  Port=3
  Abs : Abs  ZeroCross=off
  Brake Pressure Control : Subsystem  VariantControlMode=Label  Variant=on  LabelModeActiveChoice=0
  Constant1 : Constant  Value=-20
  Gain3 : Gain
  Integrator2 : Integrator  LimitOutput=on  UpperSaturationLimit=1  LowerSaturationLimit=0
  Saturation : Saturate  UpperLimit=1  LowerLimit=0  ZeroCross=off
  Switch1 : Switch  Criteria=u2 > Threshold  Threshold=.1
  Vector Concatenate2 : Concatenate  NumInputs=4
  PCmd : Outport  VectorParamsAs1DForOutWhenUnconnected=off
  wires:
  Switch1/1 -> Integrator2/1
  BrkCmd/1 -> Gain3/1, Switch1/2
  Vector Concatenate2/1 -> Brake Pressure Control/1(Pref)  "Reference P"
  Abs/1 -> Saturation/1
  xdot/1 -> Brake Pressure Control/2(xdot)
  Integrator2/1 -> Vector Concatenate2/1, Vector Concatenate2/2, Vector Concatenate2/3, Vector Concatenate2/4
  kappa/1 -> Abs/1
  Brake Pressure Control/1(PCmd) -> PCmd/1
  Saturation/1 -> Brake Pressure Control/3(<Kappa>)  "Kappa"
  Gain3/1 -> Switch1/1
  Constant1/1 -> Switch1/3

== system ISReferenceApplication/Controllers1/ECU ==
  <Accel> : Inport
  Acc to Torque Request : Gain  Gain=150
  Trq Cmd : Outport  VectorParamsAs1DForOutWhenUnconnected=off
  wires:
  Acc to Torque Request/1 -> Trq Cmd/1
  <Accel>/1 -> Acc to Torque Request/1

== system ISReferenceApplication/Controllers1/Transmission Controller ==
  Acc : Inport
  EngSpd : Inport  Port=2  Unit=rad/s
  PropShaftSpd : Inport  Port=3
  10ms Function-Call Generator : simulink/Ports & Subsystems/Function-Call Generator  sample_time=0.01  numberOfIterations=1
  Data Type Conversion : DataTypeConversion
  First Order Hold : FirstOrderHold  ErrorTolerance=.1
  Rate Transition : RateTransition  Deterministic=off
  Rate Transition1 : RateTransition  Deterministic=off
  Rate Transition2 : RateTransition  Deterministic=off
  Signal Specification : SignalSpecification  Unit=rpm
  TCM : Subsystem
  Unit Conversion : UnitConversion
  Gear : Outport  VectorParamsAs1DForOutWhenUnconnected=off
  wires:
  Data Type Conversion/1 -> First Order Hold/1
  EngSpd/1 -> Unit Conversion/1
  Signal Specification/1 -> Rate Transition1/1  "EngSpd"
  Unit Conversion/1 -> Signal Specification/1
  First Order Hold/1 -> Gear/1
  Rate Transition2/1 -> TCM/3(VehSpdFdbk)
  Rate Transition1/1 -> TCM/2(EngSpd)
  PropShaftSpd/1 -> Rate Transition2/1
  Acc/1 -> Rate Transition/1
  10ms Function-Call Generator/1 -> TCM/Trigger
  Rate Transition/1 -> TCM/1(AccCmd)
  TCM/1(Gear Select) -> Data Type Conversion/1

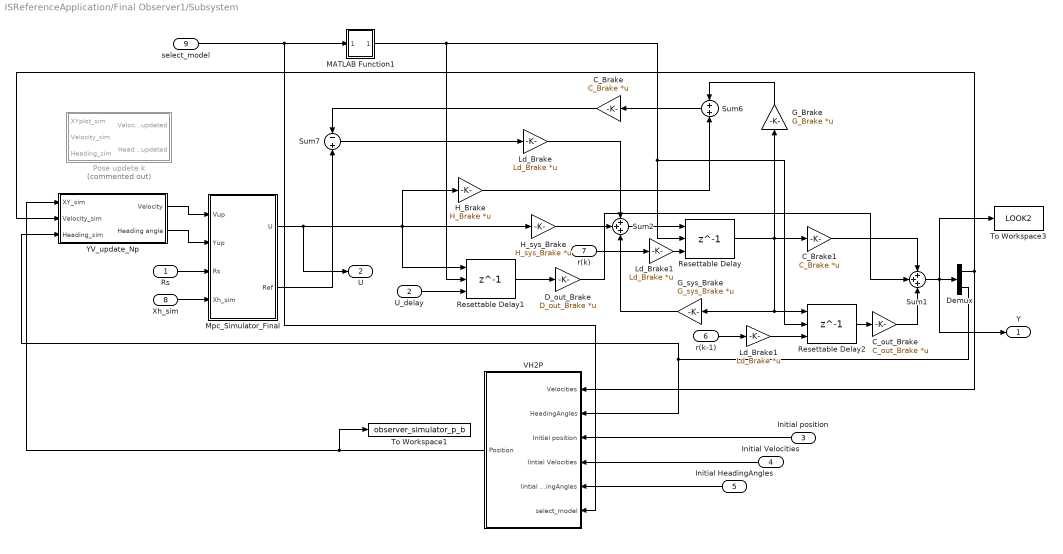
== system ISReferenceApplication/Final Observer1/Subsystem ==
  Rs : Inport
  U_delay : Inport  Port=2
  Initial position : Inport  Port=3
  Initial Velocities : Inport  Port=4
  Initial HeadingAngles : Inport  Port=5
  r(k-1) : Inport  Port=6
  r(k) : Inport  Port=7
  Xh_sim : Inport  Port=8
  select_model : Inport  Port=9
  C_Brake : Gain  Gain=C_Brake  Multiplication=Matrix(K*u) (u vector)
  C_Brake1 : Gain  Gain=C_Brake  Multiplication=Matrix(K*u) (u vector)
  C_out_Brake : Gain  Gain=C_out_Brake  Multiplication=Matrix(K*u) (u vector)
  D_out_Brake : Gain  Gain=D_out_Brake  Multiplication=Matrix(K*u) (u vector)
  Demux : Demux  Outputs=2
  G_Brake : Gain  Gain=G_Brake  Multiplication=Matrix(K*u) (u vector)
  G_sys_Brake : Gain  Gain=G_sys_Brake  Multiplication=Matrix(K*u) (u vector)
  H_Brake : Gain  Gain=H_Brake  Multiplication=Matrix(K*u) (u vector)
  H_sys_Brake : Gain  Gain=H_sys_Brake  Multiplication=Matrix(K*u) (u vector)
  Ld_Brake : Gain  Gain=Ld_Brake  Multiplication=Matrix(K*u) (u vector)
  Ld_Brake1 : Gain  Gain=Ld_Brake  Multiplication=Matrix(K*u) (u vector)
  "Ld_Brake1 " : Gain  Gain=Ld_Brake  Multiplication=Matrix(K*u) (u vector)
  MATLAB Function1 : MATLAB Function  TreatAsAtomicUnit=on
  Mpc_Simulator_Final : Subsystem
  Pose updete k : Subsystem  Commented=on
  Resettable Delay : Delay  DelayLength=1  InitialConditionSource=Input port  ExternalReset=Rising  SampleTime=Ts
      settings: InputPortMap=u0,r5,p4
  Resettable Delay1 : Delay  DelayLength=1  InitialConditionSource=Input port  ExternalReset=Rising  SampleTime=Ts
      settings: InputPortMap=u0,r5,p4
  Resettable Delay2 : Delay  DelayLength=1  InitialConditionSource=Input port  ExternalReset=Rising  SampleTime=Ts
      settings: InputPortMap=u0,r5,p4
  Sum1 : Sum  Inputs=+++
  Sum2 : Sum  Inputs=+++
  Sum6 : Sum
  Sum7 : Sum  Inputs=-+
  To Workspace1 : ToWorkspace  VariableName=observer_simulator_p_b  SampleTime=Ts
  To Workspace3 : ToWorkspace  VariableName=LOOK2  SampleTime=Ts
  VH2P : Subsystem
  YV_update_Np : Subsystem  TreatAsAtomicUnit=on
  Y : Outport  VectorParamsAs1DForOutWhenUnconnected=off
  U : Outport  Port=2  VectorParamsAs1DForOutWhenUnconnected=off
  wires:
  U_delay/1 -> Resettable Delay1/3
  Initial position/1 -> VH2P/3(Initial position)
  Mpc_Simulator_Final/1(U) -> U/1, Resettable Delay1/1, H_sys_Brake/1, H_Brake/1
  Resettable Delay/1 -> G_sys_Brake/1, Resettable Delay2/1, C_Brake1/1, G_Brake/1
  Sum7/1 -> Ld_Brake/1
  C_Brake1/1 -> Sum1/1
  Rs/1 -> Mpc_Simulator_Final/3(Rs)
  Demux/1 -> YV_update_Np/2(Velocity_sim), VH2P/1(Velocities)
  Demux/2 -> YV_update_Np/3(Heading_sim), VH2P/2(HeadingAngles)
  Resettable Delay1/1 -> D_out_Brake/1
  Ld_Brake/1 -> Sum2/1
  Initial Velocities/1 -> VH2P/4(Iintial Velocities)
  D_out_Brake/1 -> Sum1/2
  YV_update_Np/1(Velocity) -> Mpc_Simulator_Final/1(Vup)
  r(k)/1 -> "Ld_Brake1 "/1
  Resettable Delay2/1 -> C_out_Brake/1
  G_sys_Brake/1 -> Sum2/3
  r(k-1)/1 -> Ld_Brake1/1
  C_Brake/1 -> Sum7/1
  Sum2/1 -> Resettable Delay/1
  VH2P/1(Position) -> YV_update_Np/1(XY_sim), To Workspace1/1
  YV_update_Np/2(Heading angle) -> Mpc_Simulator_Final/2(Yup)
  Xh_sim/1 -> Mpc_Simulator_Final/4(Xh_sim)
  "Ld_Brake1 "/1 -> Resettable Delay/3
  Initial HeadingAngles/1 -> VH2P/5(Iintial HeadingAngles)
  G_Brake/1 -> Sum6/1
  H_Brake/1 -> Sum6/2
  C_out_Brake/1 -> Sum1/3
  Sum1/1 -> Y/1, To Workspace3/1, Demux/1
  Sum6/1 -> C_Brake/1
  Mpc_Simulator_Final/2(Ref) -> Sum7/2
  H_sys_Brake/1 -> Sum2/2
  Ld_Brake1/1 -> Resettable Delay2/3
  select_model/1 -> VH2P/6(select_model), MATLAB Function1/1(select_model)
  MATLAB Function1/1(tri) -> Resettable Delay1/2, Resettable Delay2/2, Resettable Delay/2

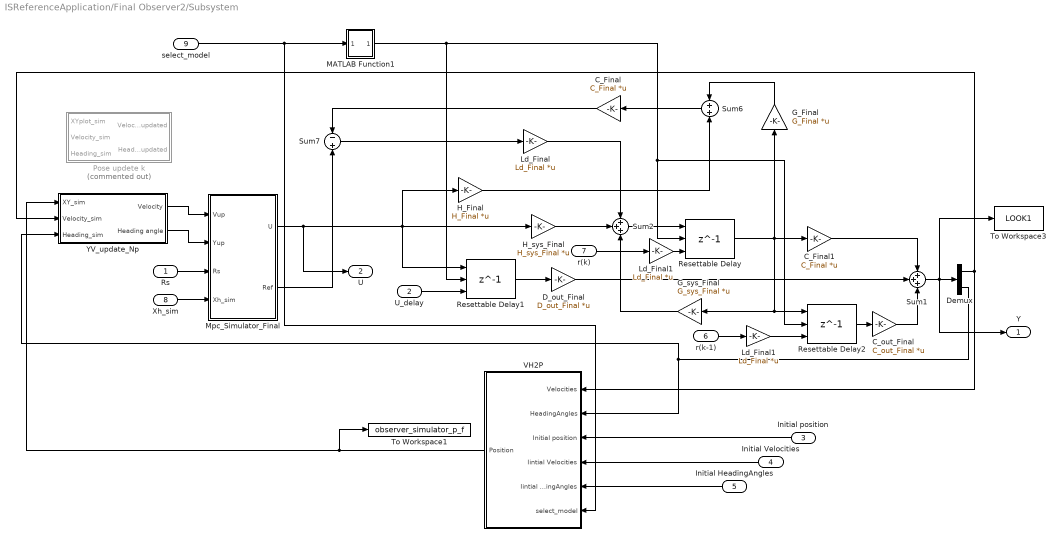
== system ISReferenceApplication/Final Observer2/Subsystem ==
  Rs : Inport
  U_delay : Inport  Port=2
  Initial position : Inport  Port=3
  Initial Velocities : Inport  Port=4
  Initial HeadingAngles : Inport  Port=5
  r(k-1) : Inport  Port=6
  r(k) : Inport  Port=7
  Xh_sim : Inport  Port=8
  select_model : Inport  Port=9
  C_Final : Gain  Gain=C_Final  Multiplication=Matrix(K*u) (u vector)
  C_Final1 : Gain  Gain=C_Final  Multiplication=Matrix(K*u) (u vector)
  C_out_Final : Gain  Gain=C_out_Final  Multiplication=Matrix(K*u) (u vector)
  D_out_Final : Gain  Gain=D_out_Final  Multiplication=Matrix(K*u) (u vector)
  Demux : Demux  Outputs=2
  G_Final : Gain  Gain=G_Final  Multiplication=Matrix(K*u) (u vector)
  G_sys_Final : Gain  Gain=G_sys_Final  Multiplication=Matrix(K*u) (u vector)
  H_Final : Gain  Gain=H_Final  Multiplication=Matrix(K*u) (u vector)
  H_sys_Final : Gain  Gain=H_sys_Final  Multiplication=Matrix(K*u) (u vector)
  Ld_Final : Gain  Gain=Ld_Final  Multiplication=Matrix(K*u) (u vector)
  Ld_Final1 : Gain  Gain=Ld_Final  Multiplication=Matrix(K*u) (u vector)
  "Ld_Final1 " : Gain  Gain=Ld_Final  Multiplication=Matrix(K*u) (u vector)
  MATLAB Function1 : MATLAB Function  TreatAsAtomicUnit=on
  Mpc_Simulator_Final : Subsystem
  Pose updete k : Subsystem  Commented=on
  Resettable Delay : Delay  DelayLength=1  InitialConditionSource=Input port  ExternalReset=Rising  SampleTime=Ts
      settings: InputPortMap=u0,r5,p4
  Resettable Delay1 : Delay  DelayLength=1  InitialConditionSource=Input port  ExternalReset=Rising  SampleTime=Ts
      settings: InputPortMap=u0,r5,p4
  Resettable Delay2 : Delay  DelayLength=1  InitialConditionSource=Input port  ExternalReset=Rising  SampleTime=Ts
      settings: InputPortMap=u0,r5,p4
  Sum1 : Sum  Inputs=+++
  Sum2 : Sum  Inputs=+++
  Sum6 : Sum
  Sum7 : Sum  Inputs=-+
  To Workspace1 : ToWorkspace  VariableName=observer_simulator_p_f  SampleTime=Ts
  To Workspace3 : ToWorkspace  VariableName=LOOK1  SampleTime=Ts
  VH2P : Subsystem
  YV_update_Np : Subsystem  TreatAsAtomicUnit=on
  Y : Outport  VectorParamsAs1DForOutWhenUnconnected=off
  U : Outport  Port=2  VectorParamsAs1DForOutWhenUnconnected=off
  wires:
  MATLAB Function1/1(tri) -> Resettable Delay/2, Resettable Delay2/2, Resettable Delay1/2
  select_model/1 -> MATLAB Function1/1(select_model), VH2P/6(select_model)
  Ld_Final1/1 -> Resettable Delay2/3
  H_sys_Final/1 -> Sum2/2
  Mpc_Simulator_Final/2(Ref) -> Sum7/2
  Sum6/1 -> C_Final/1
  Sum1/1 -> Demux/1, To Workspace3/1, Y/1
  C_out_Final/1 -> Sum1/3
  H_Final/1 -> Sum6/2
  G_Final/1 -> Sum6/1
  Initial HeadingAngles/1 -> VH2P/5(Iintial HeadingAngles)
  "Ld_Final1 "/1 -> Resettable Delay/3
  Xh_sim/1 -> Mpc_Simulator_Final/4(Xh_sim)
  YV_update_Np/2(Heading angle) -> Mpc_Simulator_Final/2(Yup)
  VH2P/1(Position) -> To Workspace1/1, YV_update_Np/1(XY_sim)
  Sum2/1 -> Resettable Delay/1
  C_Final/1 -> Sum7/1
  r(k-1)/1 -> Ld_Final1/1
  G_sys_Final/1 -> Sum2/3
  Resettable Delay2/1 -> C_out_Final/1
  r(k)/1 -> "Ld_Final1 "/1
  YV_update_Np/1(Velocity) -> Mpc_Simulator_Final/1(Vup)
  D_out_Final/1 -> Sum1/2
  Initial Velocities/1 -> VH2P/4(Iintial Velocities)
  Ld_Final/1 -> Sum2/1
  Resettable Delay1/1 -> D_out_Final/1
  Demux/2 -> VH2P/2(HeadingAngles), YV_update_Np/3(Heading_sim)
  Demux/1 -> VH2P/1(Velocities), YV_update_Np/2(Velocity_sim)
  Rs/1 -> Mpc_Simulator_Final/3(Rs)
  C_Final1/1 -> Sum1/1
  Sum7/1 -> Ld_Final/1
  Resettable Delay/1 -> G_Final/1, C_Final1/1, Resettable Delay2/1, G_sys_Final/1
  Mpc_Simulator_Final/1(U) -> H_Final/1, H_sys_Final/1, Resettable Delay1/1, U/1
  Initial position/1 -> VH2P/3(Initial position)
  U_delay/1 -> Resettable Delay1/3

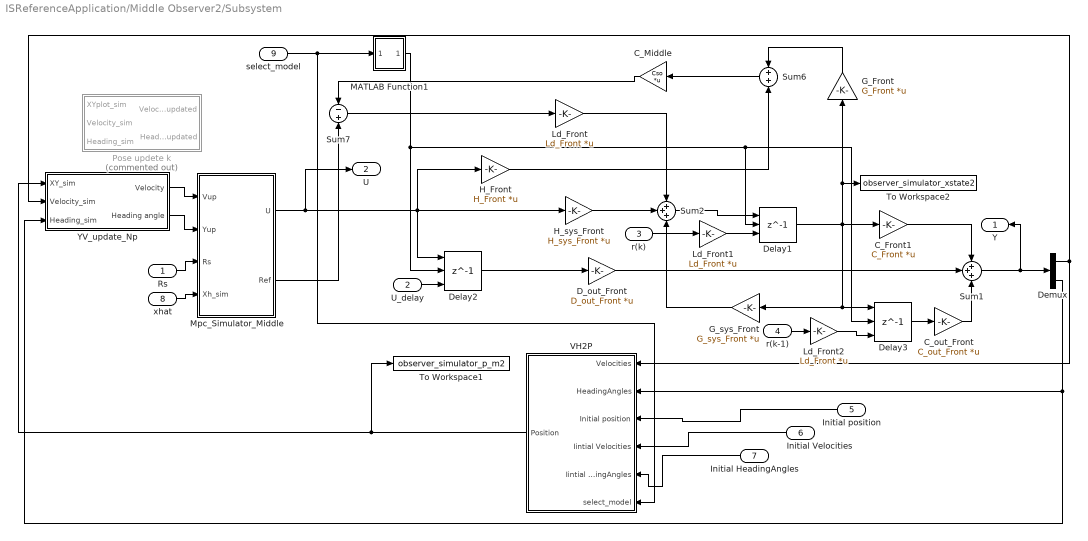
== system ISReferenceApplication/Middle Observer2/Subsystem ==
  Rs : Inport
  U_delay : Inport  Port=2
  r(k) : Inport  Port=3
  r(k-1) : Inport  Port=4
  Initial position : Inport  Port=5
  Initial Velocities : Inport  Port=6
  Initial HeadingAngles : Inport  Port=7
  xhat : Inport  Port=8
  select_model : Inport  Port=9
  C_Front1 : Gain  Gain=C_Front  Multiplication=Matrix(K*u) (u vector)
  C_Middle : Gain  Gain=Cso  Multiplication=Matrix(K*u) (u vector)
  C_out_Front : Gain  Gain=C_out_Front  Multiplication=Matrix(K*u) (u vector)
  D_out_Front : Gain  Gain=D_out_Front  Multiplication=Matrix(K*u) (u vector)
  Delay1 : Delay  DelayLength=1  InitialConditionSource=Input port  InitialCondition=0  ExternalReset=Rising  SampleTime=Ts
      settings: InputPortMap=u0,r5,p4
  Delay2 : Delay  DelayLength=1  InitialConditionSource=Input port  InitialCondition=0  ExternalReset=Rising  SampleTime=Ts
      settings: InputPortMap=u0,r5,p4
  Delay3 : Delay  DelayLength=1  InitialConditionSource=Input port  InitialCondition=0  ExternalReset=Rising  SampleTime=Ts
      settings: InputPortMap=u0,r5,p4
  Demux : Demux  Outputs=2
  G_Front : Gain  Gain=G_Front  Multiplication=Matrix(K*u) (u vector)
  G_sys_Front : Gain  Gain=G_sys_Front  Multiplication=Matrix(K*u) (u vector)
  H_Front : Gain  Gain=H_Front  Multiplication=Matrix(K*u) (u vector)
  H_sys_Front : Gain  Gain=H_sys_Front  Multiplication=Matrix(K*u) (u vector)
  Ld_Front : Gain  Gain=Ld_Front  Multiplication=Matrix(K*u) (u vector)
  Ld_Front1 : Gain  Gain=Ld_Front  Multiplication=Matrix(K*u) (u vector)
  Ld_Front2 : Gain  Gain=Ld_Front  Multiplication=Matrix(K*u) (u vector)
  MATLAB Function1 : MATLAB Function  TreatAsAtomicUnit=on
  Mpc_Simulator_Middle : Subsystem
  Pose updete k : Subsystem  Commented=on
  Sum1 : Sum  Inputs=+++
  Sum2 : Sum  Inputs=+++
  Sum6 : Sum
  Sum7 : Sum  Inputs=-+
  To Workspace1 : ToWorkspace  VariableName=observer_simulator_p_m2  SampleTime=Ts
  To Workspace2 : ToWorkspace  VariableName=observer_simulator_xstate2  SampleTime=Ts
  VH2P : Subsystem
  YV_update_Np : Subsystem  TreatAsAtomicUnit=on
  Y : Outport  VectorParamsAs1DForOutWhenUnconnected=off
  U : Outport  Port=2  VectorParamsAs1DForOutWhenUnconnected=off
  wires:
  MATLAB Function1/1(tri) -> Delay2/2, Delay1/2, Delay3/2
  select_model/1 -> MATLAB Function1/1(select_model), VH2P/6(select_model)
  Initial HeadingAngles/1 -> VH2P/5(Iintial HeadingAngles)
  Initial Velocities/1 -> VH2P/4(Iintial Velocities)
  Ld_Front2/1 -> Delay3/3
  r(k-1)/1 -> Ld_Front2/1
  U_delay/1 -> Delay2/3
  Ld_Front1/1 -> Delay1/3
  r(k)/1 -> Ld_Front1/1
  YV_update_Np/1(Velocity) -> Mpc_Simulator_Middle/1(Vup)
  xhat/1 -> Mpc_Simulator_Middle/4(Xh_sim)
  YV_update_Np/2(Heading angle) -> Mpc_Simulator_Middle/2(Yup)
  C_Front1/1 -> Sum1/1
  Delay2/1 -> D_out_Front/1
  D_out_Front/1 -> Sum1/2
  Sum6/1 -> C_Middle/1
  Sum1/1 -> Demux/1, Y/1
  H_Front/1 -> Sum6/2
  Delay1/1 -> C_Front1/1, Delay3/1, G_sys_Front/1, G_Front/1, To Workspace2/1
  Demux/1 -> VH2P/1(Velocities), YV_update_Np/2(Velocity_sim)
  VH2P/1(Position) -> To Workspace1/1, YV_update_Np/1(XY_sim)
  Delay3/1 -> C_out_Front/1
  G_sys_Front/1 -> Sum2/3
  H_sys_Front/1 -> Sum2/2
  Mpc_Simulator_Middle/1(U) -> H_Front/1, H_sys_Front/1, Delay2/1, U/1
  C_Middle/1 -> Sum7/1
  G_Front/1 -> Sum6/1
  C_out_Front/1 -> Sum1/3
  Rs/1 -> Mpc_Simulator_Middle/3(Rs)
  Mpc_Simulator_Middle/2(Ref) -> Sum7/2
  Sum7/1 -> Ld_Front/1
  Ld_Front/1 -> Sum2/1
  Demux/2 -> VH2P/2(HeadingAngles), YV_update_Np/3(Heading_sim)
  Sum2/1 -> Delay1/1
  Initial position/1 -> VH2P/3(Initial position)
